simulink model "closecircuit"  (R2022b)
settings: Solver=ode45  StartTime=0.0  StopTime=0.002  MaxStep=1e-8  RelTol=1e-3
undefined symbols (not defined in the file or in its folder): plecs
libraries: plecslib_extras2 x1, simulink x1
settings Model: Creator=qawse  LastModifiedBy=qawse
settings DataIOCC: ReturnWorkspaceOutputs=off

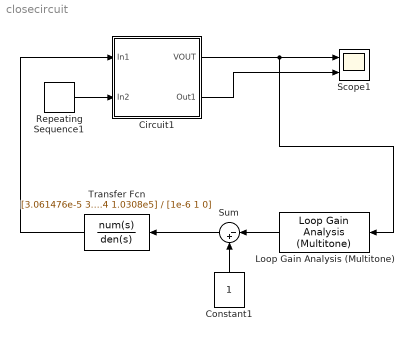
== system closecircuit ==
  Circuit1 : Subsystem  LoadFcn=plecs('sl', 200);  InitFcn=plecs('sl', 214);  StartFcn=plecs('sl', 208);  StopFcn=plecs('sl', 209);  mask(PlecsCircuit){PLECSData=<binary blob, 3024 chars, not shown>}
      mask prompts: PLECSData "PLECS Data (Do not delete or modify!)"
      mask init:
      | % PLACE CUSTOM INITIALIZATIONS ABOVE
      | % DO NOT REMOVE
      | plecs('sl', 215);
      | % DO NOT REMOVE
      settings: CopyFcn=plecs('sl', 203);  DeleteFcn=plecs('sl', 205);  UndoDeleteFcn=plecs('sl', 206);  PreSaveFcn=plecs('sl', 211);  PostSaveFcn=plecs('sl', 201);  NameChangeFcn=plecs('sl', 210);  DestroyFcn=plecs('sl', 207);  PreCopyFcn=plecs('sl', 216);  OpenFcn=plecs('sl', 202);  ErrorFcn=plerrorfcn
      mask Help: web(['file:///' fullfile(plecsdoc, 'creatingacircuit.html')])
      mask Display: disp('PLECS\nCircuit')
  Constant1 : Constant
  Loop Gain Analysis (Multitone) : plecslib_extras2/Analysis Tools/Loop Gain Analysis (Multitone)  FreqRange=[100 50000]  Amplitude=1e-4  TStart=0.02  Display=final  HideScopes=off  OutputName=T  BodePlot=on
      settings: SourceProductName=PLECS Extras
  Repeating Sequence1 : simulink/Sources/Repeating Sequence  rep_seq_t=[0 2e-6]  rep_seq_y=[0 3]
  Scope1 : Scope  NumInputPorts=2
  Sum : Sum  Inputs=|-+
  Transfer Fcn : TransferFcn  Numerator=[3.061476e-5 3.91704 1.0308e5]  Denominator=[1e-6 1 0]
  wires:
  Constant1/1 -> Sum/2
  Sum/1 -> Transfer Fcn/1
  Repeating Sequence1/1 -> Circuit1/2(In2)
  Circuit1/2(Out1) -> Scope1/2
  Transfer Fcn/1 -> Circuit1/1(In1)
  Loop Gain Analysis (Multitone)/1 -> Sum/1
  Circuit1/1(VOUT) -> Loop Gain Analysis (Multitone)/1, Scope1/1

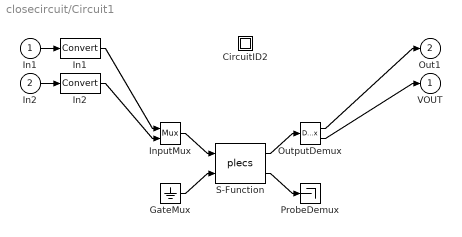
== system closecircuit/Circuit1 ==
  In1 : Inport  PortDimensions=1
  In2 : Inport  Port=2  PortDimensions=1
  " CircuitID2 " : Subsystem
  " GateMux " : Ground
  " In1 " : DataTypeConversion
  " In2 " : DataTypeConversion
  " InputMux " : Mux  Inputs=[ 1 1 ]
  " OutputDemux " : Demux  Outputs=[ 1 1 ]
  " ProbeDemux " : Terminator
  " S-Function " : S-Function  FunctionName=plecs  SFunctionDeploymentMode=off  EnableBusSupport=off
  VOUT : Outport  PortDimensions=1
  Out1 : Outport  Port=2  PortDimensions=1
  wires:
  " InputMux "/1 -> " S-Function "/1
  " GateMux "/1 -> " S-Function "/2
  " S-Function "/1 -> " OutputDemux "/1
  " S-Function "/2 -> " ProbeDemux "/1
  In1/1 -> " In1 "/1
  " In1 "/1 -> " InputMux "/1
  In2/1 -> " In2 "/1
  " In2 "/1 -> " InputMux "/2
  " OutputDemux "/1 -> Out1/1
  " OutputDemux "/2 -> VOUT/1

== system closecircuit/Circuit1/ CircuitID2  ==
